simulink model "GalvoModel_v40"  (R2013a)
settings: Solver=ode45  StartTime=0.0  StopTime=10.0  RelTol=1e-3
PostLoadFcn:
  | scopes = find_system(gcs, 'BlockType', 'Scope');
  | 
  | for i=1:length(scopes)
  |   set_param(scopes{i},'open','off');
  | end
InitFcn:
  | %JR=evalin('base',param.JR);
  | %KMT=evalin('base',param.KMT);
  | %Rc=evalin('base',param.Rc);
  | %Lc=evalin('base',param.Lc);
  | %KFR=evalin('base',param.KFR);
  | %KTB=evalin('base',param.KTB);
  | %KBM=evalin('base',param.KBM);
  | %Rsh=evalin('base',param.Rsh);
  | 
  | %JR=param.JR
  | KMT
model workspace (MATLAB code in the model file):
  | param=evalin('base','loadGalvoParam(4)')
  | evalGalvoParam(4)
  | %JR=param.JR;
  | %KMT=param.KMT;
  | %Rc=param.Rc;
  | %Lc=param.Lc;
  | %KFR=param.KFR;
  | %KTB=param.KTB;
  | %KBM=param.KBM;
  | %Rsh=param.Rsh;
undefined symbols (not defined in the file): JR, KBM, KFR, KMT, KTB, Lc, Rc, Rsh
settings Model: BufferReuse=off  Creator=mainster  LastModifiedBy=mainster
settings DataIOCC: SaveOutput=off  SaveTime=off
settings OptimizationCC: InlineParams=on  BufferReuse=off
settings DebuggingCC: InitInArrayFormatMsg=none
settings ModelReferenceCC: ModelReferenceMinAlgLoopOccurrences=on

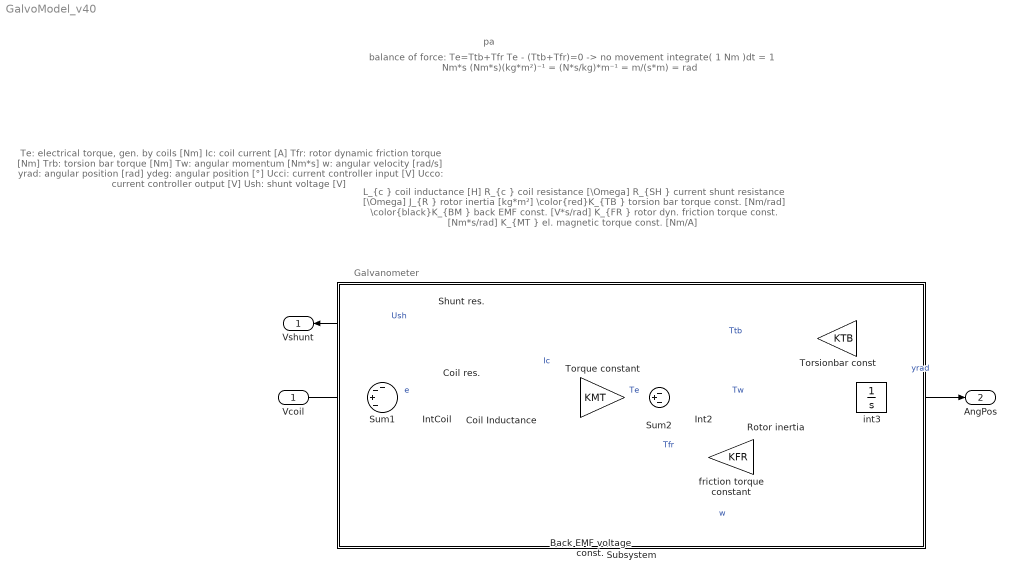
== system GalvoModel_v40 ==
  note: pa
  note: Galvanometer
  note: Te: 		electrical torque, gen. by coils		[Nm]
      |  Ic: 			coil current							[A]
      |  Tfr:		rotor dynamic friction torque 		[Nm]
      |  Trb:		torsion bar torque					[Nm]
      |  Tw:		angular momentum				[Nm*s]
      |  w:			angular velocity 					[rad/s]
      |  yrad:		angular position 					[rad]
      |  ydeg:		angular position 					[°]
      |  Ucci:		current controller input				[V]
      |  Ucco:		current controller output			[V]
      |  Ush:		shunt voltage						[V]
  note: balance of force: 	Te=Ttb+Tfr
      | 					Te - (Ttb+Tfr)=0  ->  no movement
      |
      |  integrate( 1 Nm )dt = 1 Nm*s
      |  (Nm*s)(kg*m²)⁻¹ = (N*s/kg)*m⁻¹ = m/(s*m) = rad
  note: L_{c  }	coil inductance 							[H]
      |  R_{c  }	coil resistance							[\Omega]
      |  R_{SH }	current shunt resistance				[\Omega]
      |  J_{R  }	rotor inertia 							[kg*m²]
      |  \color{red}K_{TB }	torsion bar torque const. 			[Nm/rad]
      |  \color{black}K_{BM }	back EMF const.							[V*s/rad]
      |  K_{FR }	rotor dyn. friction torque const.	[Nm*s/rad]
      |  K_{MT }	el. magnetic torque const.			[Nm/A]
  Vcoil : Inport
  Back EMF voltage const. : Gain  Gain=KBM
  Coil Inductance : Gain  Gain=1/Lc
  Coil res. : Gain  Gain=Rc
  Int2 : Integrator
  IntCoil : Integrator
  Rotor inertia : Gain  Gain=1/JR
  Shunt res. : Gain  Gain=Rsh
  Subsystem : Subsystem  RequirementInfo={} %GIDa_a4ee7dd2_92ee_443e_92b4_380bce3b8eed  mask{d=0}
      mask Display: disp('')
  Sum1 : Sum  Inputs=--+-|
  Sum2 : Sum  Inputs=-+-
  Torque constant : Gain  Gain=KMT
  Torsionbar const : Gain  Gain=KTB
  friction torque constant : Gain  Gain=KFR
  int3 : Integrator
  Vshunt : Outport
  AngPos : Outport  Port=2
  wires:
  Shunt res./1 -> Vshunt/1, Sum1/2  "Ush"
  Coil res./1 -> Sum1/1
  Vcoil/1 -> Sum1/3
  Back EMF voltage const./1 -> Sum1/4
  int3/1 -> AngPos/1, Torsionbar const/1  "yrad"
  Torque constant/1 -> Sum2/2  "Te"
  Coil Inductance/1 -> Shunt res./1, Torque constant/1, Coil res./1  "Ic"
  Torsionbar const/1 -> Sum2/1  "Ttb"
  IntCoil/1 -> Coil Inductance/1
  Sum1/1 -> IntCoil/1  "e"
  Int2/1 -> Rotor inertia/1  "Tw"
  Sum2/1 -> Int2/1
  Rotor inertia/1 -> int3/1, Back EMF voltage const./1, friction torque constant/1  "w"
  friction torque constant/1 -> Sum2/3  "Tfr"

== system GalvoModel_v40/Subsystem ==
